simulink model "Project10x2810x29"  (R2024b)
settings: Solver=ode4  StartTime=0.0  StopTime=25  FixedStep=0.001  RelTol=1e-3
model workspace (MAT data in the model file):
  A = 1
  J = 1
  b = 10
  w_0 = 1
settings Model: Creator=Joseph  LastModifiedBy=btagl

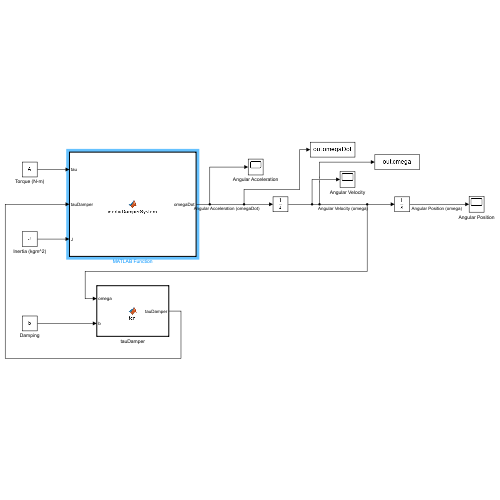
[thumbnail: Simulink's stored preview of the top-level diagram]
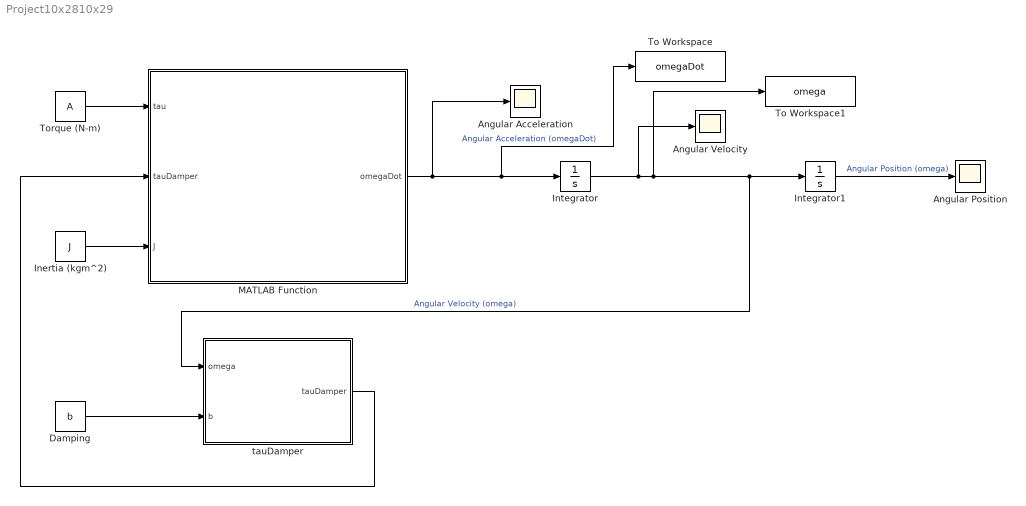
== system Project10x2810x29 ==
  Angular Acceleration : Scope
  Angular Position : Scope
  Angular Velocity : Scope
  Damping : Constant  Value=b
  Inertia (kgm^2) : Constant  Value=J
  Integrator : Integrator  InitialCondition=w_0
  Integrator1 : Integrator
  MATLAB Function : MATLAB Function  TreatAsAtomicUnit=on
  To Workspace : ToWorkspace  VariableName=omegaDot  SaveFormat=Timeseries  SampleTime=-1
  To Workspace1 : ToWorkspace  VariableName=omega  SaveFormat=Timeseries  SampleTime=-1
  Torque (N-m) : Constant  Value=A
  tauDamper : MATLAB Function  TreatAsAtomicUnit=on
  wires:
  MATLAB Function/1(omegaDot) -> Angular Acceleration/1, To Workspace/1, Integrator/1  "Angular Acceleration (omegaDot)"
  Integrator/1 -> Angular Velocity/1, tauDamper/1(omega), Integrator1/1, To Workspace1/1  "Angular Velocity (omega)"
  Integrator1/1 -> Angular Position/1  "Angular Position (omega)"
  Torque (N-m)/1 -> MATLAB Function/1(tau)
  Inertia (kgm^2)/1 -> MATLAB Function/3(J)
  Damping/1 -> tauDamper/2(b)
  tauDamper/1(tauDamper) -> MATLAB Function/2(tauDamper)

== matlab function Project10x2810x29/tauDamper ==
  data: omega input; tauDamper output; b input
function tauDamper = fcn(omega, b)

tauDamper = omega*b;

== matlab function Project10x2810x29/MATLAB Function ==
  data: tau input; omegaDot output; tauDamper input; J input
function omegaDot = inertiaDamperSystem(tau, tauDamper, J)
omegaDot = (tau-tauDamper)/J;
